simulink model "Copy_of_modelo_completo_joystick"  (R2021a)
settings: Solver=FixedStepAuto  StartTime=0.0  StopTime=inf  FixedStep=0.001  MaxStep=1e-4  RelTol=1e-3
undefined symbols (not defined in the file): bah, bat, bcx, bcy, beqhd, beqt, bw, cols_centers, cols_height, ddxmax, ddxmin, ddymax, ddymin, g, Kcy, Ksah, Ksat, Ksiah, Ksiat, Kw, lh0, max_m, Meqh, Meqt, Rd, rt, rth, Rw, sp_mass, w_mt_h, w_mt_i, xmax, xt0, yl0, yt0
libraries: simulink_extras x1, dspswit3 x1, aerolibanimutils x1, simulink x1
(part 2 of 2)

== stateflow chart Copy_of_modelo_completo_joystick/Control Level 1 - Global Supervisor Control1 ==
  state LEVEL1
    entry:
    heights = cols_height;
    centers = cols_centers;
    manual=0;
    dec = 1;
    indice=9;
    balance_deactivate = 0;
    to_where=where_;
    dc_exit = 0;
    p0=[0,0];p1=[0,0];p2=[0,0];p3=[0,0];
    p4=[0,0];p5=[0,0];p6=[0,0];p7=[0,0];
    VH_MAX=1.5,VT_MAX=4;
    %[p0,p1,p2,p3,p4,p5,p6,p7] = generate_trajectory_2(ml,VH_MAX,VT_MAX,to_where,loading,heights,centers,cycle_,indice);
    state PD_BALANCEO [parallel]
      settings: executionOrder=3
      state ACTIVATE
        balance = 1;
      state DEACTIVATE
        balance  = 0;
      (default) -> ACTIVATE
      DEACTIVATE -> ACTIVATE : [balance_deactivate == 0]
      ACTIVATE -> DEACTIVATE : [balance_deactivate == 1]
    state MOVEMENT [parallel]
      settings: executionOrder=2
      state AUTOMATIC
        state TO_SHIP
          state HOISTING_ONLY
            state INIT
            state UP
              dxt = 0;
              dlh = -VH_MAX*dec;
            state DOWN
              dxt = 0;
              dlh = VH_MAX*dec;
            (default) -> LEVEL1.MOVEMENT.AUTOMATIC.TO_SHIP.HOISTING_ONLY.INIT
            LEVEL1.MOVEMENT.AUTOMATIC.TO_SHIP.HOISTING_ONLY.INIT -> LEVEL1.MOVEMENT.AUTOMATIC.TO_SHIP.HOISTING_ONLY.DOWN [order 1] : [current_stage==5 && prev_stage==4]
            LEVEL1.MOVEMENT.AUTOMATIC.TO_SHIP.HOISTING_ONLY.INIT -> LEVEL1.MOVEMENT.AUTOMATIC.TO_SHIP.HOISTING_ONLY.UP [order 2] : [current_stage==1&& prev_stage==0]
          state INIT
          state HOISTING_AND_TROLLEY
            state UP
              dxt = VT_MAX*dec;
              dlh = -VH_MAX*dec;
            state DOWN
              dxt = 0;
              dlh = VH_MAX*dec;
            state INIT
            (default) -> LEVEL1.MOVEMENT.AUTOMATIC.TO_SHIP.HOISTING_AND_TROLLEY.INIT
            LEVEL1.MOVEMENT.AUTOMATIC.TO_SHIP.HOISTING_AND_TROLLEY.INIT -> LEVEL1.MOVEMENT.AUTOMATIC.TO_SHIP.HOISTING_AND_TROLLEY.UP [order 1] : [current_stage == 2 && prev_stage == 1]
            LEVEL1.MOVEMENT.AUTOMATIC.TO_SHIP.HOISTING_AND_TROLLEY.INIT -> LEVEL1.MOVEMENT.AUTOMATIC.TO_SHIP.HOISTING_AND_TROLLEY.DOWN [order 2] : [current_stage== 4 && prev_stage == 3]
          state TROLLEY_ONLY
            dxt = VT_MAX*dec;
            dlh = 0;
          (default) -> LEVEL1.MOVEMENT.AUTOMATIC.TO_SHIP.INIT
          LEVEL1.MOVEMENT.AUTOMATIC.TO_SHIP.INIT -> LEVEL1.MOVEMENT.AUTOMATIC.TO_SHIP.HOISTING_ONLY
          LEVEL1.MOVEMENT.AUTOMATIC.TO_SHIP.HOISTING_ONLY -> LEVEL1.MOVEMENT.AUTOMATIC.TO_SHIP.HOISTING_AND_TROLLEY : [current_stage==2 && prev_stage==1]
          LEVEL1.MOVEMENT.AUTOMATIC.TO_SHIP.HOISTING_AND_TROLLEY -> LEVEL1.MOVEMENT.AUTOMATIC.TO_SHIP.HOISTING_ONLY [order 2] : [current_stage == 5 && prev_stage == 4]
          LEVEL1.MOVEMENT.AUTOMATIC.TO_SHIP.HOISTING_AND_TROLLEY -> LEVEL1.MOVEMENT.AUTOMATIC.TO_SHIP.TROLLEY_ONLY [order 1] : [current_stage==3 && prev_stage==2]
          LEVEL1.MOVEMENT.AUTOMATIC.TO_SHIP.TROLLEY_ONLY -> LEVEL1.MOVEMENT.AUTOMATIC.TO_SHIP.HOISTING_AND_TROLLEY : [current_stage == 4 && prev_stage == 3]
        state INIT
          entry:
          [p0,p1,p2,p3,p4,p5,p6,p7] = generate_trajectory_2(ml,VH_MAX,VT_MAX,to_where,loading,heights,centers,cycle_,indice);
        state TO_DOCK
          state HOISTING_ONLY
            state UP
              dxt = 0;
              dlh = -VH_MAX*dec;
            state INIT
            state DOWN
              dxt = 0;
              dlh = VH_MAX*dec;
            (default) -> LEVEL1.MOVEMENT.AUTOMATIC.TO_DOCK.HOISTING_ONLY.INIT
            LEVEL1.MOVEMENT.AUTOMATIC.TO_DOCK.HOISTING_ONLY.INIT -> LEVEL1.MOVEMENT.AUTOMATIC.TO_DOCK.HOISTING_ONLY.UP [order 1] : [current_stage == 6 && prev_stage == 7]
            LEVEL1.MOVEMENT.AUTOMATIC.TO_DOCK.HOISTING_ONLY.INIT -> LEVEL1.MOVEMENT.AUTOMATIC.TO_DOCK.HOISTING_ONLY.DOWN [order 2] : [current_stage == 2&& prev_stage == 3]
          state INIT
          state HOISTING_AND_TROLLEY
            state UP
              dxt = -VT_MAX*dec;
              dlh = -VH_MAX*dec;
            state INIT
            state DOWN
              dxt = -VT_MAX*dec;
              dlh = VH_MAX*dec;
            (default) -> LEVEL1.MOVEMENT.AUTOMATIC.TO_DOCK.HOISTING_AND_TROLLEY.INIT
            LEVEL1.MOVEMENT.AUTOMATIC.TO_DOCK.HOISTING_AND_TROLLEY.INIT -> LEVEL1.MOVEMENT.AUTOMATIC.TO_DOCK.HOISTING_AND_TROLLEY.UP [order 2] : [current_stage == 5 && prev_stage == 6]
            LEVEL1.MOVEMENT.AUTOMATIC.TO_DOCK.HOISTING_AND_TROLLEY.INIT -> LEVEL1.MOVEMENT.AUTOMATIC.TO_DOCK.HOISTING_AND_TROLLEY.DOWN [order 1] : [current_stage == 3 && prev_stage == 4 ]
          state TROLLEY_ONLY
            during:
            dxt = -VT_MAX*dec;
            dlh = 0;
          (default) -> LEVEL1.MOVEMENT.AUTOMATIC.TO_DOCK.INIT
          LEVEL1.MOVEMENT.AUTOMATIC.TO_DOCK.INIT -> LEVEL1.MOVEMENT.AUTOMATIC.TO_DOCK.HOISTING_ONLY
          LEVEL1.MOVEMENT.AUTOMATIC.TO_DOCK.HOISTING_ONLY -> LEVEL1.MOVEMENT.AUTOMATIC.TO_DOCK.HOISTING_AND_TROLLEY : [current_stage == 5 && prev_stage == 6]
          LEVEL1.MOVEMENT.AUTOMATIC.TO_DOCK.HOISTING_AND_TROLLEY -> LEVEL1.MOVEMENT.AUTOMATIC.TO_DOCK.HOISTING_ONLY [order 1] : [current_stage == 2 && prev_stage == 3]
          LEVEL1.MOVEMENT.AUTOMATIC.TO_DOCK.HOISTING_AND_TROLLEY -> LEVEL1.MOVEMENT.AUTOMATIC.TO_DOCK.TROLLEY_ONLY [order 2] : [current_stage == 4 && prev_stage == 5]
          LEVEL1.MOVEMENT.AUTOMATIC.TO_DOCK.TROLLEY_ONLY -> LEVEL1.MOVEMENT.AUTOMATIC.TO_DOCK.HOISTING_AND_TROLLEY : [current_stage == 3 && prev_stage == 4]
        LEVEL1.MOVEMENT.AUTOMATIC.INIT -> TO_SHIP [order 1] : [current_stage == 1 && prev_stage == 0]
        (default) -> LEVEL1.MOVEMENT.AUTOMATIC.INIT
        LEVEL1.MOVEMENT.AUTOMATIC.INIT -> TO_DOCK [order 2] : [current_stage == 6 && prev_stage == 7]
      state MANUAL
        state HYBRID_MANUAL
          state TROLLEY [parallel]
            settings: executionOrder=2
            state STOP
              entry:
              dxt=0;
            state MOVE
              during:
              dxt=VT_MAX*joy_t;
            (default) -> LEVEL1.MOVEMENT.MANUAL.HYBRID_MANUAL.TROLLEY.MOVE
            LEVEL1.MOVEMENT.MANUAL.HYBRID_MANUAL.TROLLEY.STOP -> LEVEL1.MOVEMENT.MANUAL.HYBRID_MANUAL.TROLLEY.MOVE : [joy_t~=0]
            LEVEL1.MOVEMENT.MANUAL.HYBRID_MANUAL.TROLLEY.MOVE -> LEVEL1.MOVEMENT.MANUAL.HYBRID_MANUAL.TROLLEY.STOP : [joy_t==0]
          state HOISTING [parallel]
            settings: executionOrder=1
            state MOVE
              during:
              if mass_flag == 0
              dlh=VH_MAX*joy_h*0.075;
              elseif mass_flag == 1
              dlh=VH_MAX*joy_h;
              end
            state STOP
              entry:
              dlh=0;
            (default) -> LEVEL1.MOVEMENT.MANUAL.HYBRID_MANUAL.HOISTING.MOVE
            LEVEL1.MOVEMENT.MANUAL.HYBRID_MANUAL.HOISTING.STOP -> LEVEL1.MOVEMENT.MANUAL.HYBRID_MANUAL.HOISTING.MOVE : [joy_h~=0]
            LEVEL1.MOVEMENT.MANUAL.HYBRID_MANUAL.HOISTING.MOVE -> LEVEL1.MOVEMENT.MANUAL.HYBRID_MANUAL.HOISTING.STOP : [joy_h==0 ]
        (default) -> HYBRID_MANUAL
      TO_SHIP -> HYBRID_MANUAL : [current_stage == 6 && prev_stage == 5]
      (default) -> MANUAL
      HYBRID_MANUAL -> AUTOMATIC [order 1] : [manual==0 && current_stage ==  1 && prev_stage == 0 && to_where==0 && auto_mode == 1 && ( cycle_==0 || (cycle_==1 && twt==1))]
      HYBRID_MANUAL -> AUTOMATIC [order 2] : [manual==0 && current_stage == 6 && prev_stage == 7 && to_where==1 && auto_mode == 1 && ( cycle_==0 || (cycle_==1 && twt==1)) ]
      TO_DOCK -> HYBRID_MANUAL : [current_stage == 1 && prev_stage == 2]
      AUTOMATIC -> MANUAL : [(joy_t~=0 || joy_h~=0) && auto_mode==0]
    state TRAJECTORY [parallel]
      settings: executionOrder=1
      state WAITING_FOR_FLAG
      state INIT
        entry:
        [VH_MAX,VT_MAX] = calculate_vhmax(ml)
        [p0,p1,p2,p3,p4,p5,p6,p7] = generate_trajectory_2(ml,VH_MAX,VT_MAX,to_where,loading,heights,centers,cycle_,indice);
        manual=0;
      state DOUBLE_CYCLE_WAITING
        %Trayectoria manual se ejecuta
        % durante este tiempo
        during:
        [VH_MAX,VT_MAX] = calculate_vhmax(ml)
        exit:
        % detectamos el indice de columa
        indice = detect_index(x,cols_centers);
        to_where=changewhere(to_where)
        dc_exit = 1;
      state FINISH
        % Por defecto configurado para ciclo simple.
        entry:
        if cycle_ == 0
        to_where=changewhere(to_where)
        indice=changeindex(cycle_)
        manual=1;
        end
        [VH_MAX,VT_MAX] = calculate_vhmax(ml)
        [p0,p1,p2,p3,p4,p5,p6,p7] = generate_trajectory_2(ml,VH_MAX,VT_MAX,to_where,loading,heights,centers,cycle_,indice);
        exit:
        dc_exit = 0;
      state STAGE_7
        entry:
        current_stage=7;
        exit:
        prev_stage=7;
        manual=0;
      state STAGE_0
        entry:
        current_stage = 0;
        exit:
        prev_stage=0;
        manual=0;
      state STAGE_6
        entry:
        current_stage=6;
        exit:
        prev_stage=6;
      state STAGE_1
        entry:
        current_stage = 1;
        exit:
        prev_stage=1;
      state STAGE_2
        entry:
        current_stage = 2;
        exit:
        prev_stage=2;
      state STAGE_5
        entry:
        current_stage=5;
        exit:
        prev_stage=5;
      state STAGE_4
        entry:
        current_stage=4;
        exit:
        prev_stage=4;
      state STAGE_3
        entry:
        current_stage=3;
        [p4]=update_trajectory(p4,y)
        [p2]=update_p2(p2,VH_MAX)
        exit:
        prev_stage=3;
      (default) -> WAITING_FOR_FLAG
      WAITING_FOR_FLAG -> LEVEL1.TRAJECTORY.INIT : [mass_flag == 1]
      LEVEL1.TRAJECTORY.INIT -> STAGE_7 [order 2] : [y>=p7(2) && to_where == 1]
      LEVEL1.TRAJECTORY.INIT -> STAGE_0 [order 1] : [to_where == 0 && (y>=p0(2) && x>=p0(1))]
      FINISH -> DOUBLE_CYCLE_WAITING [order 3] : [cycle_ == 1 && dc_exit == 0]
      DOUBLE_CYCLE_WAITING -> FINISH : [manual_completed == 1]
      STAGE_7 -> FINISH [order 1] : [to_where == 0]
      FINISH -> STAGE_7 [order 2] : [y>=p7(2) && to_where == 1]
      FINISH -> STAGE_0 [order 1] : [y>=p0(2) && x<=p0(1) && to_where == 0 ]
      STAGE_0 -> FINISH [order 2] : [to_where == 1]
      STAGE_7 -> STAGE_6 [order 2] : [y>=p6(2)  &&  to_where == 1]
      STAGE_6 -> STAGE_7 [order 1] : [ y<=p7(2) &&  to_where == 0]
      STAGE_0 -> STAGE_1 [order 1] : [(y>=p1(2) && x>=p1(1)) &&  to_where == 0]
      STAGE_1 -> STAGE_0 [order 2] : [ y<=p0(2) &&  to_where == 1]
      STAGE_1 -> STAGE_2 [order 1] : [(y>=p2(2) && x>=p2(1)) &&  to_where == 0]
      STAGE_2 -> STAGE_1 [order 2] : [ to_where == 1 && (y<=p1(2) || x <= p1(1) || x<=-20)]
      STAGE_6 -> STAGE_5 [order 2] : [y>=p5(2) &&  to_where == 1]
      STAGE_5 -> STAGE_6 [order 1] : [ to_where == 0 && (y<=p6(2) || x >= p6(1) || x>=cols_centers(indice))]
      STAGE_2 -> STAGE_3 [order 1] : [((y>=p3(2)&&x>=p3(1)) || dlh_in == 0) &&  to_where == 0]
      STAGE_3 -> STAGE_2 [order 2] : [[(x<=p2(1) || y<=p2(2)) &&  to_where == 1]]
      STAGE_5 -> STAGE_4 [order 2] : [(y>=p4(2)&&x<=p4(1))  &&  to_where == 1]
      STAGE_4 -> STAGE_5 [order 1] : [(x>=p5(1) || y<=p5(2)) &&  to_where == 0]
      STAGE_3 -> STAGE_4 [order 1] : [ x>=p4(1) &&  to_where == 0]
      STAGE_4 -> STAGE_3 [order 2] : [ x<=p3(1) &&  to_where == 1]
  (default) -> LEVEL1
  data: p4_ function_input; p44 function_output; yl_ function_input; towhere function_input; where function_output; p2_ function_input; p22 function_output; v_ function_input; ml_ function_input; VH_MAX_ function_output; VT_MAX_ function_output; modo function_input; index function_output; xl function_input; index function_output; cols_centers_ function_input; ml_ function_input; VH_MAX_ function_input; VT_MAX_ function_input; to_where_ function_input; loading_ function_input; cols_height_ function_input; cols_centers_ function_input; mode function_input; p00 function_output; p11 function_output; p22 function_output; p33 function_output; p44 function_output; p55 function_output; p66 function_output; p77 function_output; index_ function_input; dlh_in input; dxt output; dlh output; y input; joy_t input; dxt_in input; joy_h input; auto_mode input; x input; prev_stage local =0; current_stage local =0; cycle_ input; twt input; p0 local; p1 local; p2 local; p3 local; p4 local; p5 local; p6 local; p7 local; cols_centers input; cols_height input; heights local; centers local; ml input; balance output; dec local; loading input; cycle local; where_ input; to_where local; manual local; indice local; VH_MAX local; VT_MAX local; balance_deactivate local; manual_completed input; dc_exit local; mass_flag input
  function p44 = update_trajectory(p4_,yl_):
    | function p44 = update_trajectory(p4_,yl_)
    | 
    | p44 = [p4_(1),yl_];
    | 
    | end
  function where=changewhere(towhere):
    | function where=changewhere(towhere)
    | if towhere==1
    |     where=0;
    | else
    |     where=1;
    | end
  function p22 = update_p2(p2_,v_):
    | function p22 = update_p2(p2_,v_)
    | 
    | p22 = [-20+((v_-1.5)/(3-1.5))*(16-13.5)+13.5,p2_(2)];
    | 
    | end
  function [VH_MAX_,VT_MAX_] = calculate_vhmax(ml_):
    | function [VH_MAX_,VT_MAX_] = calculate_vhmax(ml_)
    | % Valor de potencia constante a cumplir
    | Pconst = 65000*9.80665*1.5;
    | g = 9.80665;
    | VH_MAX_ = 0;
    | VT_MAX_= 0;
    | 
    | % Determinacion de velocidad del izaje segun masa de carga
    | if (ml_ <= 32500)
    |     VH_MAX_ = 3;
    | 
    | elseif (ml_ <= 65000)
    |     VH_MAX_ = Pconst / (ml_ * g);
    | end
    | 
    | VT_MAX_=4;
    | end % end function
  function index=changeindex(modo):
    | function index=changeindex(modo)
    | if modo==1
    |    index=8;
    | else
    |    index=9;
    | end
  function index=detect_index(xl,cols_centers_):
    | function index=detect_index(xl,cols_centers_)
    | % Detecta el indice de la columna actual
    | C_WIDTH = 2.5; % Ancho del contendor
    | index = 0;
    | for i=1:length(cols_centers_)
    |     aux = abs(xl-cols_centers_(i));
    |     if aux <= C_WIDTH
    |         index = i;
    |         break;
    |     end
    | end
    | end
  function [p00,p11,p22,p33,p44,p55,p66,p77] = generate_trajectory_2 (ml_,VH_MAX_,VT_MAX_,to_where_,loading_,cols_height_,cols_centers_,mode,index_):
    | function [p00,p11,p22,p33,p44,p55,p66,p77] = generate_trajectory_2 (ml_,VH_MAX_,VT_MAX_,to_where_,loading_,cols_height_,cols_centers_,mode,index_)
    | 
    | weight = ml_;
    | where = "to_ship";
    | plt_traj = "true";
    | cycle_type = "single";
    | operation_mode = "loading";
    | 
    | %% Renombramiento de variables 
    | 
    | if to_where_ == 0
    |     where = "to_ship";
    | else
    |     if to_where_ == 1
    |         where = "to_dock";
    |     end
    | end
    | 
    | if loading_ == 0
    |     operation_mode = "loading";
    | else 
    |     if loading_ == 1
    |         operation_mode = "unloading";
    |     end
    | end
    | 
    | if mode ==0 
    |     cycle_type = "single";
    | else
    |     if mode == 1
    |         cycle_type = "double";
    |     end
    | end
    | 
    | % Definimos dimensiones de un contendor maritimo [metros]
    | C_HEIGHT = 2.89;
    | C_WIDTH = 2.438;
    | c_weight = weight;
    | 
    | % Definimos dimensiones del barco (ship) [metros]
    | N_COLS = 9; % Cantidad de columnas del barco
    | MAX_C_OVER_DOCK= 9; % Cantidad maxima de containers sobre nivel del muelle
    | 
    | %% Comienzo de generacion de la trayectoria dependiendo de la situacion
    | %slope=atan(VH_MAX_/VT_MAX_); %pendiente
    | slope=atan(1.5/4); %pendiente
    | % Definimos el punto de inicio (p1) en el muelle con coordenadas x,y
    | p00=[-20,C_HEIGHT];
    | 
    | % Generamos un numero aleatorio que nos dice a que numero de columna debemos llevar el contenedor. Definimos asi p6.
    | 
    | % Indice de columna objetivo
    | index_goal=index_;
    | 
    | % Coordenada (x,y) de columna objetivo
    | p77=[cols_centers_(index_goal),cols_height_(index_goal)+C_HEIGHT];
    | 
    | % Generamos un vector que solo contenga las columnas a la izquierda del punto objetivo. Son los unicos puntos que importan.
    | left_cols=cols_height_(1:index_goal);
    | 
    | % Buscamos los de las columnas de mayor altura , tanto la que se encuentra mas a la izquierda como la que se encuentra mas a la
    | % derecha.
    | max=0;
    | imax_left=0;
    | imax_right=0;
    | for i=1:index_goal
    |     if left_cols(i)>=max
    |         imax_right=i;
    |         if left_cols(i)>max
    |             imax_left=i;
    |         end
    |     max=left_cols(i);
    |     end
    | end
    | 
    | %% Calculo de p3 y p2
    | 
    | % Definimos la altura de seguridad que me definira la coord y de p3.
    | % Se considera la altura de 2 contenedores para seguridad
    | H_SAFE=max+4*C_HEIGHT;
    | p55 = [p7(1),max+2*C_HEIGHT];
    | p66 = [p7(1),p7(2)+(p5(2)-p7(2))*0.7];
    | p44 = [p7(1) - 13,H_SAFE];
    | p33 = [-5,H_SAFE];
    | p22 = [p0(1),H_SAFE-12];
    | p11 = [p0(1),10];
    | 
    | 
    | switch(where)    
    |     case "to_ship"
    |         switch(operation_mode)
    |             case "loading"
    |                 % Puntos de viraje para velocidad maxima
    |                 p55 = [p7(1),max+2*C_HEIGHT];
    |                 p66 = [p7(1),p7(2)+(p5(2)-p7(2))*0.7];
    |                 p44 = [p7(1) - 13.2,H_SAFE];
    |                 p33 = [-5,H_SAFE];
    |                 p22 = [p0(1),H_SAFE-2*C_HEIGHT];
    |                 p11 = [p0(1),10];
    |             case "unloading"
    |                 p55 = [p7(1),max+2*C_HEIGHT];
    |                 p66 = [p7(1),p7(2)+(p5(2)-p7(2))*0.7];
    |                 p44 = [p7(1) - 13.2,H_SAFE];
    |                 p33 = [-5,H_SAFE];
    |                 p22 = [p0(1),H_SAFE-24];
    |                 p11 = [p0(1),10];
    |         end
    |        
    |               
    |     case "to_dock"
    |         switch(operation_mode)
    |             case "loading"
    |                 if cycle_type == "single"
    |                 p55 = [p7(1),max+2*C_HEIGHT];
    |                 p66 = [p7(1),p7(2)-(p5(2)-p7(2))*0.7];
    |                 p44 = [p7(1) + 13.2,H_SAFE];
    |                 p33 = [7,H_SAFE];
    |                 p22 = [p0(1)+16,H_SAFE-24];
    |                 p11 = [p0(1),10];    
    |                 disp("to dock loading");
    |                 else
    |                     
    |                 end
    |             case "unloading"
    |                 p55 = [p7(1),max+2*C_HEIGHT];
    |                 p66 = [p7(1),p7(2)-(p5(2)-p7(2))*0.7];
    |                 p44 = [p7(1) + 13.2,H_SAFE];
    |                 p33 = [7,H_SAFE];
    |                 p22 = [p0(1)+13.5,H_SAFE-24];
    |                 p11 = [p0(1),10];    
    |                 disp("to dock loading");
    |                
    |         end
    |         
    | end
    | 
    | 
    | end % end function
